simulink model "MSupGesamtFramework"  (R2018b)
settings: Solver=FixedStepDiscrete  StartTime=0.0  StopTime=inf  RelTol=1e-3  EnableMultiTasking=on
settings Model: EnablePacing=on  ExtModeTrigDuration=8  Creator=User  LastModifiedBy=mit081
settings SolverCC: AutoInsertRateTranBlk=on
settings DataIOCC: LimitDataPoints=on  SaveFormat=Array  SaveOutput=off  SaveTime=off
settings OptimizationCC: DefaultUnderspecifiedDataType=single  ExpressionDepthLimit=2147483647  LifeSpan=1  MaxStackSize=512
settings DebuggingCC: UnderspecifiedInitializationDetection=Classic  MergeDetectMultiDrivingBlocksExec=none  SolverPrmCheckMsg=warning  StateNameClashWarn=warning  SFUnexpectedBacktrackingDiag=warning  SFNoUnconditionalDefaultTransitionDiag=warning  SFExecutionAtInitializationDiag=none
settings HardwareCC: ProdBitPerChar=16  ProdBitPerInt=16  ProdBitPerPointer=32  ProdBitPerSizeT=32  ProdBitPerPtrDiffT=32  ProdLargestAtomicInteger=Integer  ProdLargestAtomicFloat=None  ProdWordSize=16  ProdLongLongMode=on  ProdHWDeviceType=Texas Instruments->C2000  TargetBitPerChar=16  TargetBitPerInt=16  TargetLargestAtomicInteger=Integer  TargetIntDivRoundTo=Zero  TargetEndianess=LittleEndian  TargetWordSize=16  TargetHWDeviceType=Texas Instruments->C2000  ProdEqTarget=off
settings ModelReferenceCC: PropagateSignalLabelsOutOfModel=off
settings SFSimCC: SimCustomSourceCode="#include \"i2c_reset.c\""  SimCustomHeaderCode="#include \"i2c_reset.h\""  SimUseLocalCustomCode=off  MATLABDynamicMemAlloc=off
settings RTWCC: SystemTargetFile=ert.tlc  HardwareBoard=TI Delfino F2833x  TemplateMakefile=ert_default_tmf  RTWUseLocalCustomCode=off  RTWUseSimCustomCode=on  CustomSourceCode="#include \"i2c_reset.c\""  CustomHeaderCode="#include \"i2c_reset.h\""  Toolchain=Texas Instruments Code Composer Studio (C2000)
settings CodeAppCC: IgnoreCustomStorageClasses=off  CustomSymbolStrType=$N$R$M  StateflowObjectComments=on  InternalIdentifier=Classic
settings ERTTargetCC: CodeReplacementLibrary=TI C28x  MultiwordLength=2048  ParMdlRefBuildCompliant=off  CPPClassGenCompliant=off  ConvertIfToSwitch=off  SuppressUnreachableDefaultCases=off
settings ConfigComp: CovMetricSettings=dw  CovHtmlReporting=on  CovSaveCumulativeToWorkspaceVar=on  CovSaveSingleToWorkspaceVar=on  CovExternalEMLEnable=off

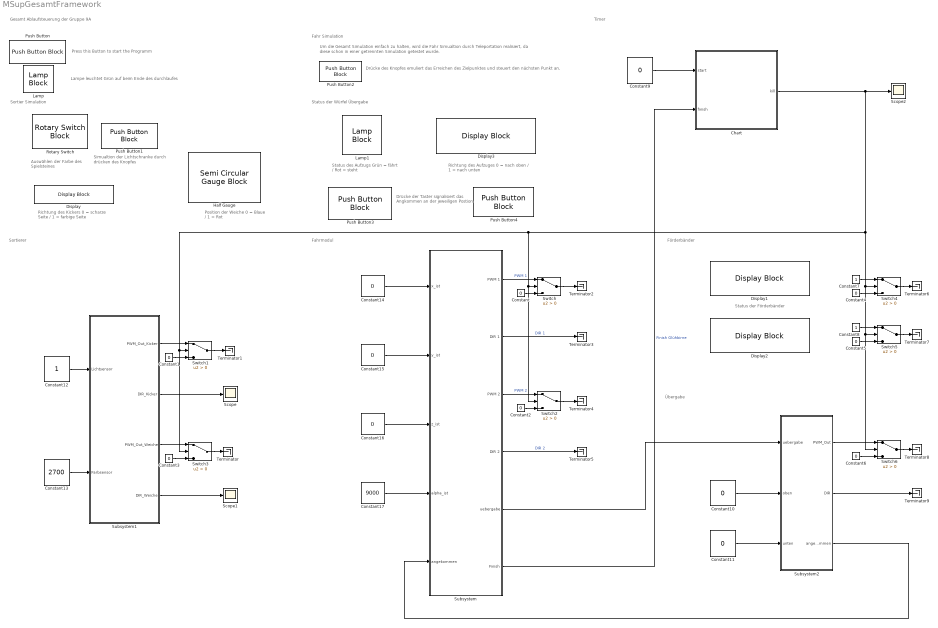
== system MSupGesamtFramework ==
  note: Drücke der Taster signalisiert
      | das Angkommen an der
      | jeweiligen Postion
  note: Drücke des Knopfes emuliert das Erreichen des Zielpunktes und steuert den nächsten
      | Punkt an.
  note: Um die Gesamt Simulation einfach zu halten, wird die Fahr Simualtion durch Teleportation realisiert,
      | da diese schon in einer getrennten Simulation getestet wurde.
  note: Fahr Simulation
  note: Richtung des Aufzuges
      | 0 = nach oben / 1 = nach unten
  note: Status des Aufzugs
      | Grün = fährt / Rot = steht
  note: Status der Würfel Übergabe
  note: Status der Förderbänder
  note: Lampe leuchtet Grün auf beim Ende des durchlaufes
  note: Position der Weiche
      | 0 = Blaue  / 1 = Rot
  note: Richtung des Kickers
      | 0 = scharze Seite / 1 = farbige Seite
  note: Simualtion der Lichtschranke
      | durch drücken des Knopfes
  note: Auswählen der Farbe
      | des Spielsteines
  note: Sortier Simulation
  note: Press this Button to start the Programm
  note: Gesamt Ablaufsteuerung der Gruppe 9A
  note: Übergabe
  note: Timer
  note: Förderbänder
  note: Fahrmodul
  note: Sortierer
  Chart : Stateflow chart  TreatAsAtomicUnit=on
  Constant{,1..6,9..11,14..16} (13 alike) : Constant  Value=0
  Constant12 : Constant
  Constant13 : Constant  Value=2700
  Constant17 : Constant  Value=9000
  Constant7 : Constant
  Constant8 : Constant
  Display : DisplayBlock  WebBlockId=362  LabelPosition=Hide
  Display1 : DisplayBlock  WebBlockId=382  LabelPosition=Hide
  Display2 : DisplayBlock  WebBlockId=384  LabelPosition=Hide
  Display3 : DisplayBlock  WebBlockId=389  LabelPosition=Hide
  Half Gauge : SemiCircularGaugeBlock  WebBlockId=365  ScaleMax=1
  Lamp : LampBlock  WebBlockId=380
  Lamp1 : LampBlock  WebBlockId=387
  Push Button : PushButtonBlock  WebBlockId=352  ButtonText=Start Button
  Push Button1 : PushButtonBlock  WebBlockId=360  ButtonText=Lichtschranke  OnValue=0
  Push Button2 : PushButtonBlock  WebBlockId=397
  Push Button3 : PushButtonBlock  WebBlockId=401  ButtonText=Taster Oben
  Push Button4 : PushButtonBlock  WebBlockId=402  ButtonText=Taster Unten
  Rotary Switch : RotarySwitchBlock  WebBlockId=357
      settings: Values={{'Rot', 'Blau', 'Schwarz'}, [400 1600 2700]}
  Scope : Scope
  Scope1 : Scope
  Scope2 : Scope
  Subsystem : Subsystem
  Subsystem1 : Subsystem
  Subsystem2 : Subsystem
  Switch{,1..6} (7 alike) : Switch  Criteria=u2 > Threshold
  Terminator{,1..9} (10 alike) : Terminator
  wires:
  Subsystem1/2(DIR_Kicker) -> Scope/1
  Subsystem1/3(PWM_Out_Weiche) -> Switch3/1
  Constant12/1 -> Subsystem1/1(Lichtsensor)
  Subsystem1/4(DIR_Weiche) -> Scope1/1
  Subsystem1/1(PWM_Out_Kicker) -> Switch1/1
  Subsystem/3(PWM 2) -> Switch2/1  "PWM 2"
  Subsystem/6(Finish) -> Chart/2(finish)  "Finish Glühbirne"
  Subsystem/4("DIR 2 ") -> Terminator5/1  "DIR 2"
  Subsystem/1(PWM 1) -> Switch/1  "PWM 1"
  Subsystem/2("DIR 1 ") -> Terminator3/1  "DIR 1"
  Constant13/1 -> Subsystem1/2(Farbsensor)
  Switch/1 -> Terminator2/1
  Constant/1 -> Switch/3
  Constant2/1 -> Switch2/3
  Switch2/1 -> Terminator4/1
  Constant1/1 -> Switch1/3
  Constant3/1 -> Switch3/3
  Switch1/1 -> Terminator1/1
  Switch3/1 -> Terminator/1
  Constant4/1 -> Switch4/3
  Switch4/1 -> Terminator6/1
  Constant5/1 -> Switch5/3
  Switch5/1 -> Terminator7/1
  Constant6/1 -> Switch6/3
  Switch6/1 -> Terminator8/1
  Chart/1(kill) -> Scope2/1, Switch2/2, Switch/2, Switch1/2, Switch3/2, Switch6/2, Switch5/2, Switch4/2
  Constant7/1 -> Switch4/1
  Constant8/1 -> Switch5/1
  Constant9/1 -> Chart/1(start)
  Subsystem2/1(PWM_Out) -> Switch6/1
  Subsystem/5(uebergabe) -> Subsystem2/1(uebergabe)
  Subsystem2/2(DIR) -> Terminator9/1
  Constant10/1 -> Subsystem2/2(oben)
  Constant11/1 -> Subsystem2/3(unten)
  Subsystem2/3(angekommen) -> Subsystem/5(angekommen)
  Constant14/1 -> Subsystem/1(x_ist)
  Constant15/1 -> Subsystem/2(y_ist)
  Constant16/1 -> Subsystem/3(z_ist)
  Constant17/1 -> Subsystem/4(alpha_ist)

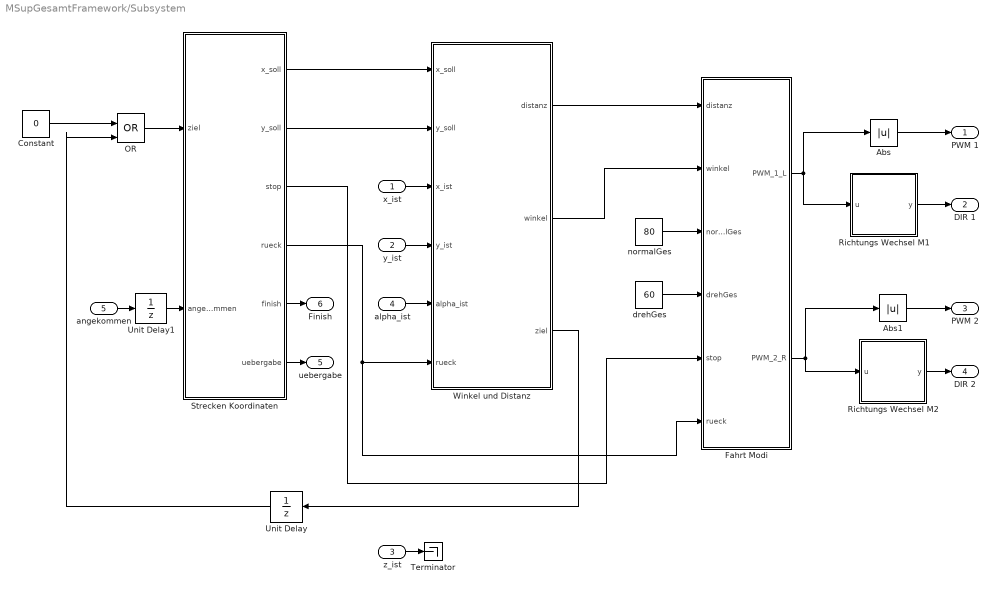
== system MSupGesamtFramework/Subsystem ==
  x_ist : Inport
  y_ist : Inport  Port=2
  z_ist : Inport  Port=3
  alpha_ist : Inport  Port=4
  angekommen : Inport  Port=5
  Abs : Abs
  Abs1 : Abs
  Constant : Constant  Value=0
  Fahrt Modi : Stateflow chart  TreatAsAtomicUnit=on
  OR : Logic  Operator=OR  IconShape=distinctive  AllPortsSameDT=off  OutDataTypeStr=boolean
  "Richtungs Wechsel M1 " : MATLAB Function  TreatAsAtomicUnit=on
  Richtungs Wechsel M2 : MATLAB Function  TreatAsAtomicUnit=on
  Strecken Koordinaten : Stateflow chart  TreatAsAtomicUnit=on
  Terminator : Terminator
  Unit Delay : UnitDelay  SampleTime=-1
  Unit Delay1 : UnitDelay  SampleTime=-1
  Winkel und Distanz : MATLAB Function  TreatAsAtomicUnit=on
  "drehGes " : Constant  Value=60
  "normalGes " : Constant  Value=80
  PWM 1 : Outport
  "DIR 1 " : Outport  Port=2
  PWM 2 : Outport  Port=3
  "DIR 2 " : Outport  Port=4
  uebergabe : Outport  Port=5
  Finish : Outport  Port=6
  wires:
  z_ist/1 -> Terminator/1
  Abs/1 -> PWM 1/1
  Abs1/1 -> PWM 2/1
  "Richtungs Wechsel M1 "/1(y) -> "DIR 1 "/1
  Fahrt Modi/1(PWM_1_L) -> Abs/1, "Richtungs Wechsel M1 "/1(u)
  Richtungs Wechsel M2/1(y) -> "DIR 2 "/1
  Fahrt Modi/2(PWM_2_R) -> Abs1/1, Richtungs Wechsel M2/1(u)
  y_ist/1 -> Winkel und Distanz/4(y_ist)
  x_ist/1 -> Winkel und Distanz/3(x_ist)
  "normalGes "/1 -> Fahrt Modi/3(normalGes)
  "drehGes "/1 -> Fahrt Modi/4(drehGes)
  Winkel und Distanz/1(distanz) -> Fahrt Modi/1(distanz)
  Winkel und Distanz/2(winkel) -> Fahrt Modi/2(winkel)
  alpha_ist/1 -> Winkel und Distanz/5(alpha_ist)
  Strecken Koordinaten/1(x_soll) -> Winkel und Distanz/1(x_soll)
  Strecken Koordinaten/2(y_soll) -> Winkel und Distanz/2(y_soll)
  Winkel und Distanz/3(ziel) -> Unit Delay/1
  Unit Delay/1 -> OR/2
  Strecken Koordinaten/3(stop) -> Fahrt Modi/5(stop)
  Strecken Koordinaten/4(rueck) -> Winkel und Distanz/6(rueck), Fahrt Modi/6(rueck)
  Strecken Koordinaten/5(finish) -> Finish/1
  Strecken Koordinaten/6(uebergabe) -> uebergabe/1
  angekommen/1 -> Unit Delay1/1
  Unit Delay1/1 -> Strecken Koordinaten/2(angekommen)
  OR/1 -> Strecken Koordinaten/1(ziel)
  Constant/1 -> OR/1

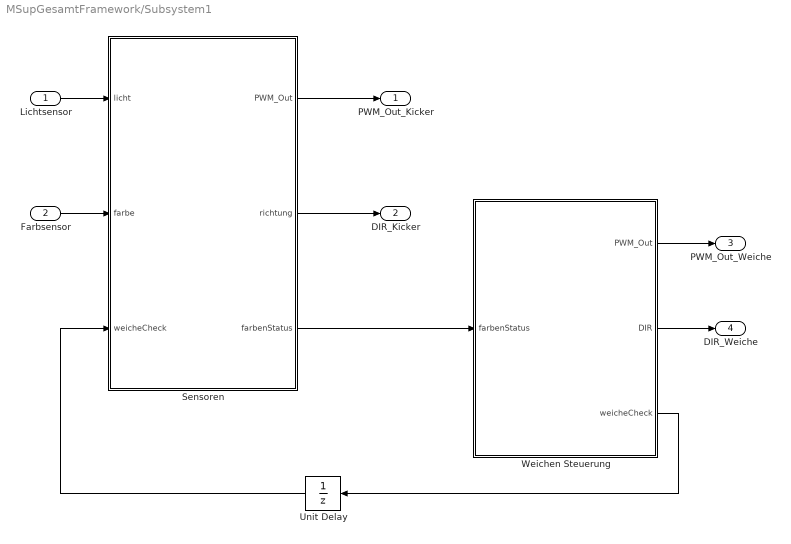
== system MSupGesamtFramework/Subsystem1 ==
  Lichtsensor : Inport
  Farbsensor : Inport  Port=2
  Sensoren : Stateflow chart  TreatAsAtomicUnit=on
  Unit Delay : UnitDelay  SampleTime=-1
  Weichen Steuerung : Stateflow chart  TreatAsAtomicUnit=on
  PWM_Out_Kicker : Outport
  DIR_Kicker : Outport  Port=2
  PWM_Out_Weiche : Outport  Port=3
  DIR_Weiche : Outport  Port=4
  wires:
  Lichtsensor/1 -> Sensoren/1(licht)
  Farbsensor/1 -> Sensoren/2(farbe)
  Sensoren/1(PWM_Out) -> PWM_Out_Kicker/1
  Sensoren/2(richtung) -> DIR_Kicker/1
  Weichen Steuerung/1(PWM_Out) -> PWM_Out_Weiche/1
  Weichen Steuerung/2(DIR) -> DIR_Weiche/1
  Sensoren/3(farbenStatus) -> Weichen Steuerung/1(farbenStatus)
  Unit Delay/1 -> Sensoren/3(weicheCheck)
  Weichen Steuerung/3(weicheCheck) -> Unit Delay/1

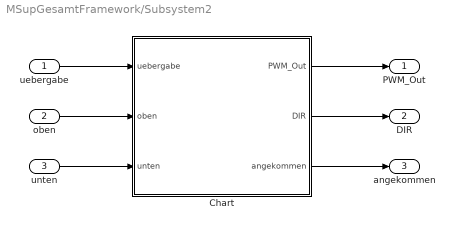
== system MSupGesamtFramework/Subsystem2 ==
  uebergabe : Inport
  oben : Inport  Port=2
  unten : Inport  Port=3
  Chart : Stateflow chart  TreatAsAtomicUnit=on
  PWM_Out : Outport
  DIR : Outport  Port=2
  angekommen : Outport  Port=3
  wires:
  Chart/1(PWM_Out) -> PWM_Out/1
  Chart/2(DIR) -> DIR/1
  uebergabe/1 -> Chart/1(uebergabe)
  oben/1 -> Chart/2(oben)
  unten/1 -> Chart/3(unten)
  Chart/3(angekommen) -> angekommen/1

== stateflow chart MSupGesamtFramework/Subsystem1/Sensoren ==
  state wartenkurz
  state warten
    en:
    PWM_Out = 0;
  state warten3
  state SchwarzOderBunt
  state Schwarz
    PWM_Out = 80;
    richtung = 0;
  state Farbe
  state blau
    en:
    farbenStatus = 0;
  state rot
    en:
    farbenStatus = 1;
  state warten4
  state Bunt
    PWM_Out = 80;
    richtung = 1;
  Schwarz -> wartenkurz : [licht == 1]
  Bunt -> wartenkurz : [licht ==1]
  wartenkurz -> warten : after(30,msec)
  (default) -> warten
  warten -> warten3 : [licht == 0]
  warten3 -> SchwarzOderBunt : after(0.2,sec)
  SchwarzOderBunt -> Schwarz [order 2] : [farbe > 2200]
  SchwarzOderBunt -> Farbe [order 1] : [farbe < 2200]
  Farbe -> blau [order 1] : [farbe > 1000]
  Farbe -> rot [order 2] : [farbe < 1000]
  rot -> warten4
  blau -> warten4
  warten4 -> Bunt : [weicheCheck == 0]
  data: licht input; PWM_Out output; richtung output; farbenStatus output; farbe input; weicheCheck input

== stateflow chart MSupGesamtFramework/Subsystem/Fahrt Modi ==
  state LinksDrehen
    entry:
    PWM_1_L = -drehGes;
    PWM_2_R = drehGes;
  state RechtsDrehen
    entry:
    PWM_1_L = drehGes;
    PWM_2_R = -drehGes;
  state Stehen
    entry:
    PWM_1_L = 0;
    PWM_2_R = 0;
  state GeradeausFahren
    entry:
    PWM_1_L = normalGes;
    PWM_2_R = normalGes;
  state Rueckwaerts
    entry:
    PWM_1_L = -drehGes;
    PWM_2_R = -drehGes;
  LinksDrehen -> RechtsDrehen [order 2] : [winkel < -10]
  RechtsDrehen -> LinksDrehen [order 2] : [winkel > 10]
  LinksDrehen -> Stehen [order 1] : [(winkel > -10 & winkel <10)||stop == 1||distanz < 300]
  Stehen -> LinksDrehen [order 2] : [winkel > 10 & stop==0]
  RechtsDrehen -> Stehen [order 1] : [(winkel > -10 & winkel < 10) || stop == 1||distanz < 300 ]
  Stehen -> RechtsDrehen [order 3] : [winkel < -10 & stop==0]
  (default) -> Stehen
  GeradeausFahren -> Stehen : [winkel < -10 || winkel > 10|| stop==1]
  Stehen -> GeradeausFahren [order 1] : [winkel > -10 & winkel < 10 & stop == 0 & rueck ==0]
  Stehen -> Rueckwaerts [order 4] : [winkel > -10 & winkel < 10 & stop == 0 & rueck == 1]
  Rueckwaerts -> Stehen : [winkel < -10 || winkel > 10|| stop==1]
  data: PWM_1_L output; PWM_2_R output; distanz input; winkel input; normalGes input; drehGes input; stop input; rueck input

== stateflow chart MSupGesamtFramework/Chart ==
  state warten
    kill = 1;
  state Anfang
    en:
    kill = 0;
  state Ende
    en:
    kill = 1;
  (default) -> warten
  warten -> Anfang : [start == 1]
  Anfang -> Ende [order 2] : [finish == 1]
  Anfang -> Ende [order 1] : after(175,sec)
  data: start input; kill output; finish input

== matlab function MSupGesamtFramework/Subsystem/Richtungs Wechsel M1  ==
  data: u input; y output
function y = fcn(u)
if u > 0
    y = 0;
else
    y = 1;
end

== matlab function MSupGesamtFramework/Subsystem/Richtungs Wechsel M2 ==
  data: u input; y output
function y = fcn(u)
    if u > 0
        y = 0;
    else
        y = 1;
    end

== stateflow chart MSupGesamtFramework/Subsystem/Strecken Koordinaten ==
  state Position2
    entry:
    x_soll = 4350;
    y_soll = 7800;
    stop = 0;
    rueck = 0;
  state Position4
    entry:
    x_soll = 7900;
    y_soll = 4060;
    stop = 0;
    rueck = 0;
  state Position5
    entry:
    x_soll = 10170;
    y_soll = 4916;
    stop = 0;
    rueck = 1;
  state Ziel
    entry:
    x_soll = 8550;
    y_soll = -2150;
    stop = 0;
    rueck = 0;
  state Stop
    entry:
    stop = 1;
    finish = 1;
  state Uebergabe
    entry:
    uebergabe = 1;
    stop = 1;
    exit:
    uebergabe = 0;
  (default) -> Position2
  Position2 -> Position4 : [ziel== 1]
  Position5 -> Uebergabe : [ziel == 1]
  Position4 -> Position5 : [ziel == 1]
  Uebergabe -> Ziel : [angekommen == 1]
  Ziel -> Stop : [ziel ==1]
  data: x_soll output; y_soll output; ziel input boolean; stop output; rueck output; finish output; uebergabe output; angekommen input

== matlab function MSupGesamtFramework/Subsystem/Winkel und Distanz ==
  data: x_soll input; distanz output; y_soll input; x_ist input; y_ist input; alpha_ist input; winkel output; ziel output; rueck input
function [distanz, winkel, ziel] = fcn(x_soll, y_soll, x_ist, y_ist, alpha_ist, rueck)
    
    % Realtive Position der Ziel Koordinaten
    x_dif = x_soll - x_ist;
    y_dif = y_soll - y_ist;
    distanz = sqrt(x_dif^2 + y_dif^2);
    winkelVor = rad2deg(atan(y_dif/x_dif));
    
    % Drehwinkel Bestimmung
    if x_dif < 0
        winkelVor = winkelVor + 180;
    else
        if y_dif < 0
            winkelVor = winkelVor + 360;
        end
    end
    % Rückwärts Funktion
    if rueck == 1
        winkelVor = winkelVor + 180;
        if winkelVor > 360
            winkelVor = winkelVor -360;
        end
    end
    
    % rechnet aktuellen Winkel mit ein
    winkelVor = winkelVor - alpha_ist/10;
    
    % bestimmt kürzere Drehdistanz
    if winkelVor > 175 
        winkelVor = winkelVor - 360;
    end
    % Winkel wird ausgegebn
    winkel = winkelVor; 
    
    % checkt ob die nächste Koordinate angefahren werden kann
    if distanz < 300
        ziel = 1;
    else
        ziel = 0;
    end

== stateflow chart MSupGesamtFramework/Subsystem1/Weichen Steuerung ==
  state linksdrehen
    en:
    PWM_Out = 50;
    DIR = 0;
    weicheCheck = 1;
  state blau
    en:
    weicheCheck = 0;
    PWM_Out = 0;
  state rot
    en:
    weicheCheck = 0;
    PWM_Out = 0;
  state rechtsdrehen
    en:
    PWM_Out = 50;
    DIR = 1;
    weicheCheck = 1;
  linksdrehen -> blau : after(0.18,sec)
  rot -> linksdrehen : [farbenStatus == 0]
  (default) -> blau
  blau -> rechtsdrehen : [farbenStatus == 1]
  rechtsdrehen -> rot : after(0.18,sec)
  data: farbenStatus input; PWM_Out output; DIR output; weicheCheck output single

== stateflow chart MSupGesamtFramework/Subsystem2/Chart ==
  state warten
    en:
    PWM_Out = 0;
    DIR = 0;
    angekommen = 0;
  state hochFahren
    en:
    PWM_Out = 100;
    DIR = 0;
  state oben
    en:
    PWM_Out = 0;
    DIR = 0;
  state runterFahren
    en:
    PWM_Out = 100;
    DIR = 1;
    angekommen = 1;
  state unten
    en:
    PWM_Out = 0;
    DIR = 0;
  (default) -> warten
  warten -> hochFahren : [uebergabe == 1]
  hochFahren -> oben : [oben == 1]
  oben -> runterFahren : after(1,sec)
  runterFahren -> unten : [unten == 1]
  data: uebergabe input; PWM_Out output; DIR output; oben input; unten input; angekommen output
